simulink model "LQR_control"  (R2022b)
settings: Solver=VariableStepAuto  StartTime=0.0  StopTime=10.0  RelTol=1e-3
undefined symbols (not defined in the file or in its folder): A, B, C, D, J
settings Model: Creator=samue  LastModifiedBy=samue

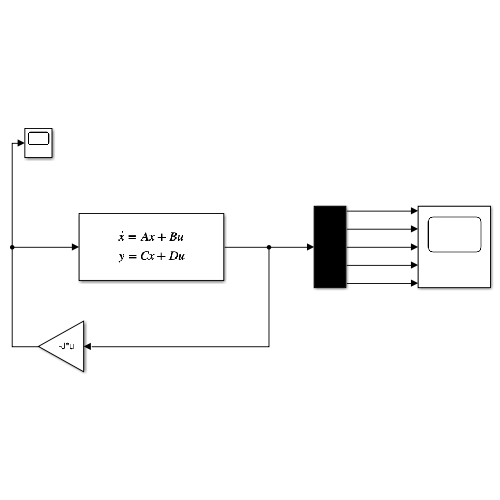
[thumbnail: Simulink's stored preview of the top-level diagram]
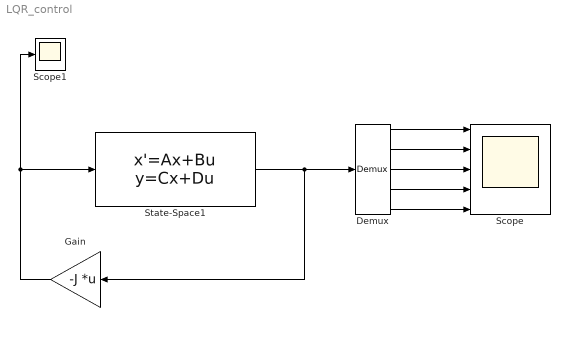
== system LQR_control ==
  Demux : Demux  Outputs=5
  Gain : Gain  Gain=-J  Multiplication=Matrix(K*u)
  Scope : Scope  NumInputPorts=5
  Scope1 : Scope
  State-Space1 : StateSpace  A=A  B=B  C=C  D=D  InitialCondition=[-1,0,0.5,0,0]
  wires:
  Demux/1 -> Scope/1
  Demux/2 -> Scope/2
  Demux/3 -> Scope/3
  Demux/4 -> Scope/4
  Demux/5 -> Scope/5
  State-Space1/1 -> Gain/1, Demux/1
  Gain/1 -> State-Space1/1, Scope1/1
